simulink model "corrector"  (R2018b)
settings: Solver=FixedStepDiscrete  StartTime=0.0  StopTime=10.0  RelTol=1e-3
libraries: simulink x1
settings Model: Creator=jayakumarav  LastModifiedBy=hiterd

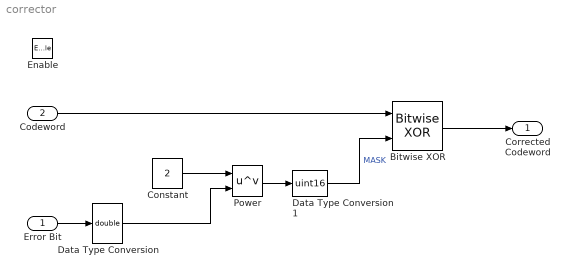
== system corrector ==
  Error Bit : Inport  OutDataTypeStr=uint16
  Codeword : Inport  Port=2
  Enable : EnablePort  OutDataTypeStr=boolean
  Bitwise XOR : simulink/Logic and Bit Operations/Bitwise Operator  logicop=XOR  UseBitMask=off  NumInputPorts=2  BitMask=bin2dec('11011001')  BitMaskRealWorld=Stored Integer
  Constant : Constant  Value=2  OutDataTypeStr=double
  Data Type Conversion : DataTypeConversion  OutDataTypeStr=double
  Data Type Conversion1 : DataTypeConversion  OutDataTypeStr=uint16
  Power : Math  Operator=pow  SaturateOnIntegerOverflow=on
  Corrected Codeword : Outport
  wires:
  Bitwise XOR/1 -> Corrected Codeword/1
  Codeword/1 -> Bitwise XOR/1
  Error Bit/1 -> Data Type Conversion/1
  Power/1 -> Data Type Conversion1/1
  Data Type Conversion1/1 -> Bitwise XOR/2  "MASK"
  Constant/1 -> Power/1
  Data Type Conversion/1 -> Power/2
